simulink model "Quadrotor_model"  (R2018a)
settings: Solver=ode45  StartTime=0.0  StopTime=tSpan  RelTol=1e-3  EnableMultiTasking=on
values from neighbouring files (symbols this model uses):
  a1 = 16.235    [QuadrotorConstants.m]    (also in QuadrotorConstants.mat; TuningParameters.mat)
  a2 = 17.912    [QuadrotorConstants.m]    (also in QuadrotorConstants.mat; TuningParameters.mat)
  a3 = 17.914    [QuadrotorConstants.m]    (also in QuadrotorConstants.mat; TuningParameters.mat)
  a4 = 18.161    [QuadrotorConstants.m]    (also in QuadrotorConstants.mat; TuningParameters.mat)
  angSatLimit = 250    [QuadrotorConstants.m]    (also in QuadrotorConstants.mat; TuningParameters.mat)
  b1 = -0.5036    [QuadrotorConstants.m]    (also in QuadrotorConstants.mat; TuningParameters.mat)
  b2 = -12.728    [QuadrotorConstants.m]    (also in QuadrotorConstants.mat; TuningParameters.mat)
  b3 = -6.5646    [QuadrotorConstants.m]    (also in QuadrotorConstants.mat; TuningParameters.mat)
  b4 = -7.4637    [QuadrotorConstants.m]    (also in QuadrotorConstants.mat; TuningParameters.mat)
  bb = 2.6846e-07    [QuadrotorConstants.m]    (also in QuadrotorConstants.mat; TuningParameters.mat)
  c = 0.0002    [QuadrotorConstants.m]    (also in QuadrotorConstants.mat; TuningParameters.mat)
  c_mi_x = 1.70    (= 1.7)    [QuadrotorConstants.m]    (also in QuadrotorConstants.mat; TuningParameters.mat)
  c_mi_y = 1.70    (= 1.7)    [QuadrotorConstants.m]    (also in QuadrotorConstants.mat; TuningParameters.mat)
  c_mi_z = 0.40    (= 0.4)    [QuadrotorConstants.m]    (also in QuadrotorConstants.mat; TuningParameters.mat)
  co_x = 1.7    [QuadrotorConstants.m]    (also in QuadrotorConstants.mat; TuningParameters.mat)
  co_y = 1.7    [QuadrotorConstants.m]    (also in QuadrotorConstants.mat; TuningParameters.mat)
  co_z = 3    [QuadrotorConstants.m]    (also in QuadrotorConstants.mat; TuningParameters.mat)
  d = 0.0071    [QuadrotorConstants.m]    (also in QuadrotorConstants.mat; TuningParameters.mat)
  d_omega_R10 = V1_WP    [InitialConditions.m]    (also in TuningParameters.mat = 0.286149195881)
  d_omega_R20 = V2_WP    [InitialConditions.m]    (also in TuningParameters.mat = 0.941828505757)
  d_omega_R30 = V3_WP    [InitialConditions.m]    (also in TuningParameters.mat = 0.597668426656)
  d_omega_R40 = V4_WP    [InitialConditions.m]    (also in TuningParameters.mat = 0.639046979523)
  dd = 2.4481e-03    (= 0.0024481)    [QuadrotorConstants.m]    (also in QuadrotorConstants.mat; TuningParameters.mat)
  dfi_0 = 0    [InitialConditions.m]    (also in TuningParameters.mat)
  disturbancePhi = 0    [runMain.m]
  disturbancePsi = 0    [runMain.m]
  disturbanceTheta = 0    [runMain.m]
  disturbancex = 0    [runMain.m]
  disturbancey = 0    [runMain.m]
  disturbancez = 0    [runMain.m]
  dpsi_0 = 0    [InitialConditions.m]    (also in TuningParameters.mat)
  dtheta_0 = 0    [InitialConditions.m]    (also in TuningParameters.mat)
  dx_0 = 0    [InitialConditions.m]    (also in TuningParameters.mat)
  dy_0 = 0    [InitialConditions.m]    (also in TuningParameters.mat)
  dz_0 = 5    [InitialConditions.m]    (also in TuningParameters.mat)
  f = 5e-6    (= 5e-06)    [QuadrotorConstants.m]    (also in QuadrotorConstants.mat; TuningParameters.mat; animateQuadrotor.m = getframe; animateQuadrotorConstant.m = getframe)
  fi_0 = pi    (= 3.14159265359)    [InitialConditions.m]    (also in TuningParameters.mat)
  g = 0.0008    [QuadrotorConstants.m]    (also in QuadrotorConstants.mat; TuningParameters.mat)
  ga = 9.807    [QuadrotorConstants.m]    (also in QuadrotorConstants.mat; TuningParameters.mat)
  h = -0.0282    [QuadrotorConstants.m]    (also in QuadrotorConstants.mat; TuningParameters.mat)
  Ixx = 2.1385*1    (= 2.1385)    [QuadrotorConstants.m]    (also in QuadrotorConstants.mat; TuningParameters.mat)
  Iyy = Ixx    (= 2.1385)    [QuadrotorConstants.m]    (also in QuadrotorConstants.mat; TuningParameters.mat)
  Izz = 3.7479*1    (= 3.7479)    [QuadrotorConstants.m]    (also in QuadrotorConstants.mat; TuningParameters.mat)
  Jr = 4.86851*0.1    (= 0.486851)    [QuadrotorConstants.m]    (also in QuadrotorConstants.mat; TuningParameters.mat)
  L = 0.422    [QuadrotorConstants.m]    (also in QuadrotorConstants.mat; TuningParameters.mat)
  lambda_phi = 50/kd_phi    (= 5)    [TuningParameters.m]    (also in TuningParameters.mat)
  lambda_psi = 50/kd_psi    (= 5)    [TuningParameters.m]    (also in TuningParameters.mat)
  lambda_theta = 50/kd_theta    (= 5)    [TuningParameters.m]    (also in TuningParameters.mat)
  lambda_z = 50/kd_z    (= 5)    [TuningParameters.m]    (also in TuningParameters.mat)
  m = 2.1    [QuadrotorConstants.m]    (also in QuadrotorConstants.mat; TuningParameters.mat)
  psi_0 = 0    [InitialConditions.m]    (also in TuningParameters.mat)
  Tau = 0.1    [QuadrotorConstants.m]    (also in QuadrotorConstants.mat; TuningParameters.mat)
  theta_0 = 0    [InitialConditions.m]    (also in TuningParameters.mat)
  x_0 = 0    [InitialConditions.m]    (also in TuningParameters.mat)
  y_0 = 0    [InitialConditions.m]    (also in TuningParameters.mat)
  z_0 = 10    [InitialConditions.m]    (also in TuningParameters.mat)
undefined symbols (not defined in the file or in its folder): sigbuilder_block
settings Model: Creator=Jake  LastModifiedBy=mdom9
settings DataIOCC: LimitDataPoints=on  SaveFormat=Array  SignalLoggingSaveFormat=ModelDataLogs
settings OptimizationCC: InitFltsAndDblsToZero=on  LifeSpan=inf
settings DebuggingCC: SaveWithParameterizedLinksMsg=none  UnderspecifiedInitializationDetection=Classic  MergeDetectMultiDrivingBlocksExec=none  SignalResolutionControl=TryResolveAllWithWarning  MultiTaskDSMMsg=warning  MultiTaskCondExecSysMsg=none  FcnCallInpInsideContextMsg=warning  SFUnexpectedBacktrackingDiag=warning  SFNoUnconditionalDefaultTransitionDiag=warning  SFExecutionAtInitializationDiag=none
settings HardwareCC: ProdBitPerPointer=32  ProdBitPerSizeT=32  ProdBitPerPtrDiffT=32  ProdLargestAtomicFloat=None  ProdIntDivRoundTo=Undefined  ProdEndianess=Unspecified  ProdWordSize=32  ProdHWDeviceType=32-bit Generic
settings ModelReferenceCC: PropagateSignalLabelsOutOfModel=off
settings SFSimCC: SimParseCustomCode=off
settings CodeAppCC: StateflowObjectComments=on
settings GRTTargetCC: TargetFcnLib=ansi_tfl_tmw.mat  TargetLangStandard=C89/C90 (ANSI)  CombineOutputUpdateFcns=off  GRTInterface=on
settings ConfigComp: CovMetricSettings=dw  CovHtmlReporting=on  CovSaveCumulativeToWorkspaceVar=on  CovSaveSingleToWorkspaceVar=on  CovExternalEMLEnable=off
settings SimscapeCC: SimscapeNormalizeSystem=off

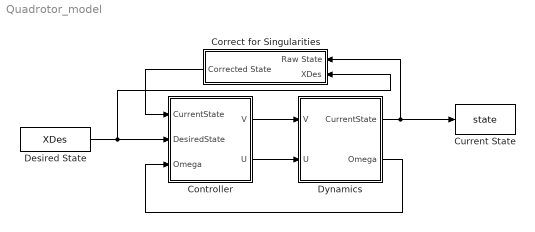
== system Quadrotor_model ==
  Controller : Subsystem
  Correct for Singularities : Subsystem
  Current State : ToWorkspace  VariableName=state  SaveFormat=Timeseries  SampleTime=-1
  Desired State : FromWorkspace  VariableName=XDes  SampleTime=0
  Dynamics : Subsystem
  wires:
  Controller/1(V) -> Dynamics/1(V)
  Dynamics/2(Omega) -> Controller/3(Omega)
  Dynamics/1("CurrentState ") -> Current State/1, Correct for Singularities/1(Raw State)
  Controller/2(U) -> Dynamics/2(U)
  Desired State/1 -> Correct for Singularities/2(XDes), Controller/2(DesiredState)
  Correct for Singularities/1(Corrected State) -> Controller/1("CurrentState ")

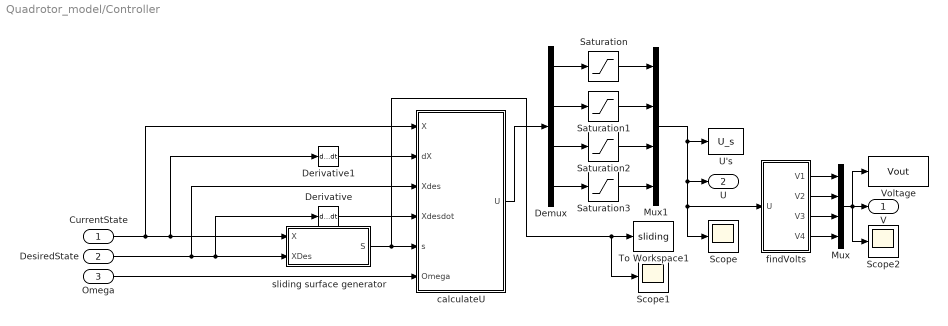
== system Quadrotor_model/Controller ==
  "CurrentState " : Inport
  DesiredState : Inport  Port=2
  Omega : Inport  Port=3
  Demux : Demux
  Derivative : Derivative
  Derivative1 : Derivative
  Mux : Mux
  Mux1 : Mux
  Saturation : Saturate  UpperLimit=60  LowerLimit=0
  Saturation1 : Saturate  UpperLimit=angSatLimit  LowerLimit=-angSatLimit
  Saturation2 : Saturate  UpperLimit=angSatLimit  LowerLimit=-angSatLimit
  Saturation3 : Saturate  UpperLimit=angSatLimit  LowerLimit=-angSatLimit
  Scope : Scope
  Scope1 : Scope
  Scope2 : Scope
  To Workspace1 : ToWorkspace  VariableName=sliding  SaveFormat=Timeseries  SampleTime=-1
  U's : ToWorkspace  VariableName=U_s  SaveFormat=Timeseries  SampleTime=-1
  Voltage : ToWorkspace  VariableName=Vout  SaveFormat=Timeseries  SampleTime=-1
  calculateU : MATLAB Function  TreatAsAtomicUnit=on
  findVolts : Subsystem
  sliding surface generator : Subsystem
  V : Outport
  U : Outport  Port=2
  wires:
  sliding surface generator/1(S) -> calculateU/5(s), Scope1/1, To Workspace1/1
  findVolts/1(V1) -> Mux/1
  findVolts/2(V2) -> Mux/2
  findVolts/3(V3) -> Mux/3
  findVolts/4(V4) -> Mux/4
  Mux/1 -> Voltage/1, Scope2/1, V/1
  Omega/1 -> calculateU/6(Omega)
  "CurrentState "/1 -> calculateU/1(X), Derivative1/1, sliding surface generator/1(X)
  DesiredState/1 -> calculateU/3(Xdes), Derivative/1, sliding surface generator/2(XDes)
  Derivative/1 -> calculateU/4(Xdesdot)
  Derivative1/1 -> calculateU/2(dX)
  Mux1/1 -> Scope/1, findVolts/1(U), U/1, U's/1
  Demux/1 -> Saturation/1
  Demux/2 -> Saturation1/1
  Demux/3 -> Saturation2/1
  Demux/4 -> Saturation3/1
  calculateU/1(U) -> Demux/1
  Saturation/1 -> Mux1/1
  Saturation1/1 -> Mux1/2
  Saturation2/1 -> Mux1/3
  Saturation3/1 -> Mux1/4

== system Quadrotor_model/Correct for Singularities ==
  Raw State : Inport
  XDes : Inport  Port=2
  "Check for singularity in phi, theta" : Subsystem
  DIsplay Uncorrected State : Subsystem
  Display Corrected State : Subsystem
  Corrected State : Outport
  wires:
  Raw State/1 -> "Check for singularity in phi, theta"/1(Current State), DIsplay Uncorrected State/1(Uncorrected State)
  "Check for singularity in phi, theta"/1("Correct State ") -> Corrected State/1, Display Corrected State/1(Corrected State)
  XDes/1 -> "Check for singularity in phi, theta"/2(XDes)

== system Quadrotor_model/Dynamics ==
  V : Inport
  U : Inport  Port=2
  Body dynamics : Subsystem
  Demux : Demux
  Demux1 : Demux
  Motor dynamics : Subsystem
  Mux : Mux  Inputs=2
  "CurrentState " : Outport
  Omega : Outport  Port=2
  wires:
  Mux/1 -> "CurrentState "/1
  V/1 -> Demux/1
  Demux/1 -> Motor dynamics/1(V1)
  Demux/2 -> Motor dynamics/2(V2)
  Demux/3 -> Motor dynamics/3(V3)
  Demux/4 -> Motor dynamics/4(V4)
  Motor dynamics/1(Omega) -> Omega/1, Body dynamics/5(Omega)
  Demux1/1 -> Body dynamics/1(U1)
  Demux1/2 -> Body dynamics/2(U2)
  Demux1/3 -> Body dynamics/3(U3)
  Demux1/4 -> Body dynamics/4(U4)
  U/1 -> Demux1/1
  Body dynamics/1(Position) -> Mux/1
  Body dynamics/2(Orientation) -> Mux/2

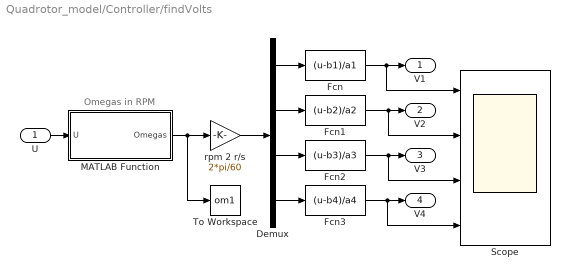
== system Quadrotor_model/Controller/findVolts ==
  note: Omegas in RPM
  U : Inport
  Demux : Demux
  Fcn : Fcn  Expr=(u-b1)/a1
  Fcn1 : Fcn  Expr=(u-b2)/a2
  Fcn2 : Fcn  Expr=(u-b3)/a3
  Fcn3 : Fcn  Expr=(u-b4)/a4
  MATLAB Function : MATLAB Function  TreatAsAtomicUnit=on
  Scope : Scope  NumInputPorts=4
  To Workspace : ToWorkspace  VariableName=om1  SaveFormat=Timeseries  SampleTime=-1
  rpm 2 r/s : Gain  Gain=2*pi/60
  V1 : Outport
  V2 : Outport  Port=2
  V3 : Outport  Port=3
  V4 : Outport  Port=4
  wires:
  Fcn3/1 -> Scope/4, V4/1
  Fcn2/1 -> Scope/3, V3/1
  Fcn1/1 -> Scope/2, V2/1
  Fcn/1 -> Scope/1, V1/1
  Demux/1 -> Fcn/1
  Demux/3 -> Fcn2/1
  Demux/2 -> Fcn1/1
  rpm 2 r/s/1 -> Demux/1
  Demux/4 -> Fcn3/1
  MATLAB Function/1(Omegas) -> To Workspace/1, rpm 2 r/s/1
  U/1 -> MATLAB Function/1(U)

== system Quadrotor_model/Controller/sliding surface generator ==
  X : Inport
  XDes : Inport  Port=2
  Add : Sum  Inputs=+++
  Derivative : Derivative
  Gain : Gain  Gain=[lambda_z lambda_phi lambda_theta lambda_psi].'
  Integrator : Integrator
  Scope : Scope
  Selector : Selector  InputPortWidth=12  IndexOptions=Index vector (dialog)  Indices=[5 7 9 11]  OutputSizes=1
  error : Sum  Inputs=-+
  S : Outport
  wires:
  Gain/1 -> Add/1
  error/1 -> Scope/1, Selector/1
  Add/1 -> S/1
  Derivative/1 -> Add/2
  Integrator/1 -> Add/3
  Selector/1 -> Integrator/1, Gain/1, Derivative/1
  X/1 -> error/1
  XDes/1 -> error/2

== system Quadrotor_model/Correct for Singularities/Check for singularity in phi, theta ==
  Current State : Inport
  XDes : Inport  Port=2
  Singularity in phi : Subsystem
  Singularity in theta : Subsystem
  "Correct State " : Outport
  wires:
  Singularity in phi/1(Modified State) -> Singularity in theta/1(Current State)
  Singularity in theta/1(Modified State) -> "Correct State "/1
  Current State/1 -> Singularity in phi/1(Current State)
  XDes/1 -> Singularity in phi/2(XDes), Singularity in theta/2(XDes)

== system Quadrotor_model/Correct for Singularities/DIsplay Uncorrected State ==
  Uncorrected State : Inport
  Constant : Constant  Value=0
  Scope1 : Scope
  Selector2 : Selector  InputPortWidth=12  IndexOptions=Index vector (dialog)  Indices=[7 9]  OutputSizes=1
  Subtract : Sum  Inputs=+-
  To Workspace1 : ToWorkspace  VariableName=rawAngles  SaveFormat=Timeseries  SampleTime=-1
  wires:
  Constant/1 -> Subtract/2
  Selector2/1 -> Subtract/1
  Subtract/1 -> Scope1/1, To Workspace1/1
  Uncorrected State/1 -> Selector2/1

== system Quadrotor_model/Correct for Singularities/Display Corrected State ==
  Corrected State : Inport
  Constant1 : Constant  Value=0
  Scope2 : Scope
  Selector1 : Selector  InputPortWidth=12  IndexOptions=Index vector (dialog)  Indices=[7 9]  OutputSizes=1
  Subtract1 : Sum  Inputs=+-
  To Workspace : ToWorkspace  VariableName=correctedAngles  SaveFormat=Timeseries  SampleTime=-1
  wires:
  Constant1/1 -> Subtract1/2
  Subtract1/1 -> To Workspace/1, Scope2/1
  Selector1/1 -> Subtract1/1
  Corrected State/1 -> Selector1/1

== system Quadrotor_model/Dynamics/Body dynamics ==
  U1 : Inport
  U2 : Inport  Port=2
  U3 : Inport  Port=3
  U4 : Inport  Port=4
  Omega : Inport  Port=5
  Mux : Mux  Inputs=6
  Pitch Stability : Subsystem
  Position Stability : Subsystem
  Roll Stability : Subsystem
  Yaw Stability : Subsystem
  Position : Outport
  Orientation : Outport  Port=2
  wires:
  U4/1 -> Yaw Stability/1(U4)
  U3/1 -> Pitch Stability/3(U3)
  U1/1 -> Position Stability/1(U1)
  U2/1 -> Roll Stability/2(U2)
  Omega/1 -> Pitch Stability/2(SumYRtrSpd), Roll Stability/1(SumXRtrSpd)
  Roll Stability/1(Phi) -> Position Stability/2(fi), Mux/1
  Pitch Stability/1(Theta) -> Position Stability/3(theta), Mux/3
  Yaw Stability/1(Psi) -> Position Stability/4(psi), Mux/5
  Roll Stability/2(dPhi) -> Mux/2, Yaw Stability/2(dPhi), Pitch Stability/1(dPhi)
  Yaw Stability/2(dPsi) -> Roll Stability/4(dPsi), Pitch Stability/4(dPsi), Mux/6
  Pitch Stability/2(dTheta) -> Yaw Stability/3(dTheta), Roll Stability/3(dTheta), Mux/4
  Position Stability/1(Position) -> Position/1
  Mux/1 -> Orientation/1

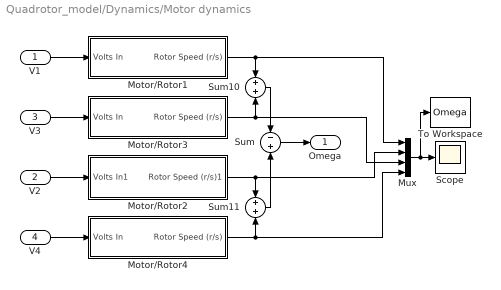
== system Quadrotor_model/Dynamics/Motor dynamics ==
  V1 : Inport
  V2 : Inport  Port=2
  V3 : Inport  Port=3
  V4 : Inport  Port=4
  Motor/Rotor1 : Subsystem
  Motor/Rotor2 : Subsystem
  Motor/Rotor3 : Subsystem
  Motor/Rotor4 : Subsystem
  Mux : Mux
  Scope : Scope
  Sum : Sum  Inputs=-+
  Sum10 : Sum  Inputs=+|+
  Sum11 : Sum  Inputs=+|+
  To Workspace : ToWorkspace  VariableName=Omega  SaveFormat=Timeseries  SampleTime=-1
  Omega : Outport
  wires:
  Sum11/1 -> Sum/2
  Sum10/1 -> Sum/1
  Motor/Rotor4/1(Rotor Speed (r/s)) -> Mux/4, Sum11/2
  Motor/Rotor3/1(Rotor Speed (r/s)) -> Mux/3, Sum10/2
  Motor/Rotor2/1(Rotor Speed (r/s)1) -> Mux/2, Sum11/1
  Motor/Rotor1/1(Rotor Speed (r/s)) -> Mux/1, Sum10/1
  Sum/1 -> Omega/1
  V1/1 -> Motor/Rotor1/1(Volts In)
  V4/1 -> Motor/Rotor4/1(Volts In)
  V3/1 -> Motor/Rotor3/1(Volts In)
  V2/1 -> Motor/Rotor2/1(Volts In1)
  Mux/1 -> To Workspace/1, Scope/1

== system Quadrotor_model/Correct for Singularities/Check for singularity in phi, theta/Singularity in phi ==
  Current State : Inport
  XDes : Inport  Port=2
  CorrectPhi : MATLAB Function  TreatAsAtomicUnit=on
  Modified State : Outport
  wires:
  Current State/1 -> CorrectPhi/1(X)
  CorrectPhi/1(newX) -> Modified State/1
  XDes/1 -> CorrectPhi/2(XDes)

== system Quadrotor_model/Correct for Singularities/Check for singularity in phi, theta/Singularity in theta ==
  Current State : Inport
  XDes : Inport  Port=2
  CorrectTheta : MATLAB Function  TreatAsAtomicUnit=on
  Modified State : Outport
  wires:
  Current State/1 -> CorrectTheta/1(X)
  CorrectTheta/1(newX) -> Modified State/1
  XDes/1 -> CorrectTheta/2(XDes)

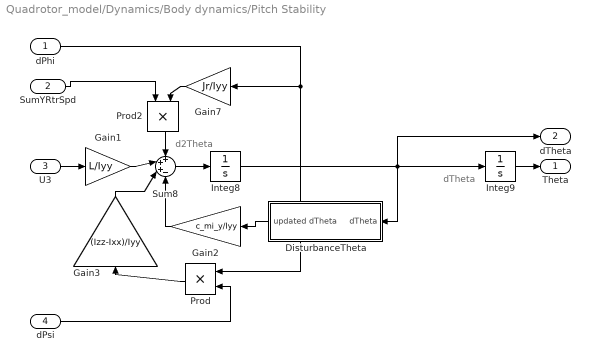
== system Quadrotor_model/Dynamics/Body dynamics/Pitch Stability ==
  note: d2Theta
  note: dTheta
  dPhi : Inport
  SumYRtrSpd : Inport  Port=2
  U3 : Inport  Port=3
  dPsi : Inport  Port=4
  DisturbanceTheta : Subsystem
  Gain1 : Gain  Gain=L/Iyy
  Gain2 : Gain  Gain=c_mi_y/Iyy
  Gain3 : Gain  Gain=(Izz-Ixx)/Iyy
  Gain7 : Gain  Gain=Jr/Iyy
  Integ8 : Integrator  InitialCondition=dtheta_0
  Integ9 : Integrator  InitialCondition=theta_0  UpperSaturationLimit=pi/2  LowerSaturationLimit=-pi/2
  Prod : Product  RndMeth=Zero
  Prod2 : Product  RndMeth=Zero
  Sum8 : Sum  Inputs=+++-
  Theta : Outport
  dTheta : Outport  Port=2
  wires:
  Gain2/1 -> Sum8/4
  dPhi/1 -> Prod/1, Gain7/1
  Integ9/1 -> Theta/1
  U3/1 -> Gain1/1
  SumYRtrSpd/1 -> Prod2/1
  dPsi/1 -> Prod/2
  Integ8/1 -> dTheta/1, DisturbanceTheta/1(dTheta), Integ9/1
  Sum8/1 -> Integ8/1
  Gain1/1 -> Sum8/2
  Gain7/1 -> Prod2/2
  Gain3/1 -> Sum8/3
  Prod/1 -> Gain3/1
  Prod2/1 -> Sum8/1
  DisturbanceTheta/1(updated dTheta) -> Gain2/1

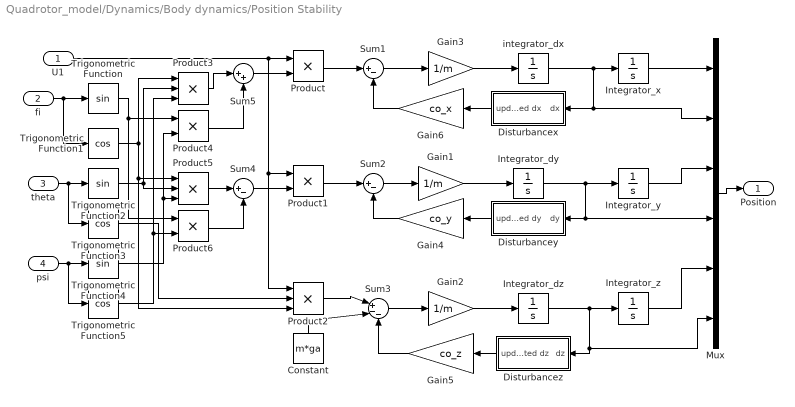
== system Quadrotor_model/Dynamics/Body dynamics/Position Stability ==
  U1 : Inport
  fi : Inport  Port=2
  theta : Inport  Port=3
  psi : Inport  Port=4
  Constant : Constant  Value=m*ga
  Disturbancex : Subsystem
  Disturbancey : Subsystem
  Disturbancez : Subsystem
  Gain1 : Gain  Gain=1/m
  Gain2 : Gain  Gain=1/m
  Gain3 : Gain  Gain=1/m
  Gain4 : Gain  Gain=co_y
  Gain5 : Gain  Gain=co_z
  Gain6 : Gain  Gain=co_x
  Integrator_dy : Integrator  InitialCondition=dy_0  LimitOutput=on  UpperSaturationLimit=1000  LowerSaturationLimit=-1000
  Integrator_dz : Integrator  InitialCondition=dz_0  LimitOutput=on  UpperSaturationLimit=1000  LowerSaturationLimit=-1000
  Integrator_x : Integrator  InitialCondition=x_0
  Integrator_y : Integrator  InitialCondition=y_0
  Integrator_z : Integrator  InitialCondition=z_0
  Mux : Mux  Inputs=6
  Product{,1,4,6} (4 alike) : Product  RndMeth=Zero
  Product2 : Product  Inputs=3  RndMeth=Zero
  Product3 : Product  Inputs=3  RndMeth=Zero
  Product5 : Product  Inputs=3  RndMeth=Zero
  Sum1 : Sum  Inputs=|+-
  Sum2 : Sum  Inputs=|+-
  Sum3 : Sum  Inputs=|+--
  Sum4 : Sum  Inputs=|+-
  Sum5 : Sum  Inputs=|++
  Trigonometric Function : Trigonometry
  Trigonometric Function1 : Trigonometry  Operator=cos
  Trigonometric Function2 : Trigonometry
  Trigonometric Function3 : Trigonometry  Operator=cos
  Trigonometric Function4 : Trigonometry
  Trigonometric Function5 : Trigonometry  Operator=cos
  integrator_dx : Integrator  InitialCondition=dx_0  LimitOutput=on  UpperSaturationLimit=1000  LowerSaturationLimit=-1000
  Position : Outport
  wires:
  Gain5/1 -> Sum3/3
  Constant/1 -> Sum3/2
  Gain4/1 -> Sum2/2
  Sum3/1 -> Gain2/1
  Gain6/1 -> Sum1/2
  Product2/1 -> Sum3/1
  Sum2/1 -> Gain1/1
  Product1/1 -> Sum2/1
  Gain2/1 -> Integrator_dz/1
  Sum1/1 -> Gain3/1
  Product/1 -> Sum1/1
  U1/1 -> Product/1, Product1/1, Product2/1
  Integrator_x/1 -> Mux/1
  integrator_dx/1 -> Integrator_x/1, Disturbancex/1(dx), Mux/2
  Integrator_dy/1 -> Integrator_y/1, Disturbancey/1(dy), Mux/4
  Integrator_dz/1 -> Integrator_z/1, Disturbancez/1(dz), Mux/6
  Gain1/1 -> Integrator_dy/1
  Gain3/1 -> integrator_dx/1
  Sum4/1 -> Product1/2
  Sum5/1 -> Product/2
  Product3/1 -> Sum5/1
  Product4/1 -> Sum5/2
  Product5/1 -> Sum4/1
  Product6/1 -> Sum4/2
  psi/1 -> Trigonometric Function4/1, Trigonometric Function5/1
  theta/1 -> Trigonometric Function2/1, Trigonometric Function3/1
  fi/1 -> Trigonometric Function/1, Trigonometric Function1/1
  Trigonometric Function/1 -> Product4/1, Product6/1
  Trigonometric Function1/1 -> Product3/1, Product5/1, Product2/3
  Trigonometric Function2/1 -> Product3/2, Product5/2
  Trigonometric Function5/1 -> Product3/3, Product6/2
  Trigonometric Function4/1 -> Product4/2, Product5/3
  Trigonometric Function3/1 -> Product2/2
  Integrator_y/1 -> Mux/3
  Integrator_z/1 -> Mux/5
  Mux/1 -> Position/1
  Disturbancez/1(updated dz) -> Gain5/1
  Disturbancey/1(updated dy) -> Gain4/1
  Disturbancex/1(updated dx) -> Gain6/1

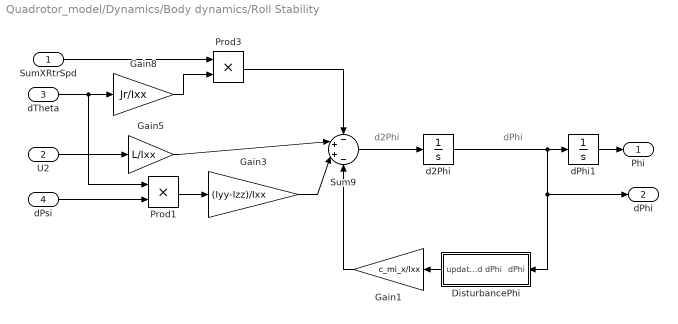
== system Quadrotor_model/Dynamics/Body dynamics/Roll Stability ==
  note: d2Phi
  note: dPhi
  SumXRtrSpd : Inport
  U2 : Inport  Port=2
  dTheta : Inport  Port=3
  dPsi : Inport  Port=4
  DisturbancePhi : Subsystem
  Gain1 : Gain  Gain=c_mi_x/Ixx
  Gain3 : Gain  Gain=(Iyy-Izz)/Ixx
  Gain5 : Gain  Gain=L/Ixx
  Gain8 : Gain  Gain=Jr/Ixx
  Prod1 : Product  RndMeth=Zero
  Prod3 : Product  RndMeth=Zero
  Sum9 : Sum  Inputs=-++-
  d2Phi : Integrator  InitialCondition=dfi_0
  dPhi1 : Integrator  InitialCondition=fi_0  UpperSaturationLimit=pi/2  LowerSaturationLimit=-pi/2
  Phi : Outport
  dPhi : Outport  Port=2
  wires:
  dPsi/1 -> Prod1/2
  dTheta/1 -> Prod1/1, Gain8/1
  Prod3/1 -> Sum9/1
  SumXRtrSpd/1 -> Prod3/1
  Gain8/1 -> Prod3/2
  dPhi1/1 -> Phi/1
  U2/1 -> Gain5/1
  d2Phi/1 -> DisturbancePhi/1(dPhi), dPhi/1, dPhi1/1
  Sum9/1 -> d2Phi/1
  Gain5/1 -> Sum9/2
  Gain1/1 -> Sum9/4
  Gain3/1 -> Sum9/3
  Prod1/1 -> Gain3/1
  DisturbancePhi/1(updated dPhi) -> Gain1/1

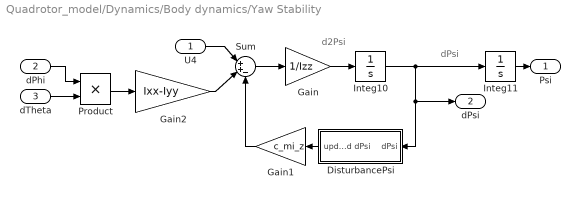
== system Quadrotor_model/Dynamics/Body dynamics/Yaw Stability ==
  note: dPsi
  note: d2Psi
  U4 : Inport
  dPhi : Inport  Port=2
  dTheta : Inport  Port=3
  DisturbancePsi : Subsystem
  Gain : Gain  Gain=1/Izz
  Gain1 : Gain  Gain=c_mi_z
  Gain2 : Gain  Gain=Ixx-Iyy
  Integ10 : Integrator  InitialCondition=dpsi_0
  Integ11 : Integrator  InitialCondition=psi_0
  Product : Product  RndMeth=Zero
  Sum : Sum  Inputs=|++-
  Psi : Outport
  dPsi : Outport  Port=2
  wires:
  Sum/1 -> Gain/1
  U4/1 -> Sum/1
  Integ11/1 -> Psi/1
  Gain/1 -> Integ10/1
  Integ10/1 -> DisturbancePsi/1(dPsi), dPsi/1, Integ11/1
  Gain1/1 -> Sum/3
  Gain2/1 -> Sum/2
  dPhi/1 -> Product/1
  dTheta/1 -> Product/2
  Product/1 -> Gain2/1
  DisturbancePsi/1(updated dPsi) -> Gain1/1

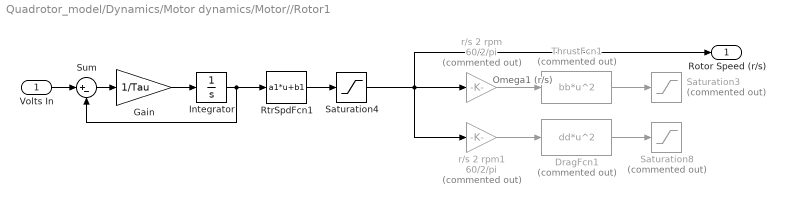
== system Quadrotor_model/Dynamics/Motor dynamics/Motor//Rotor1 ==
  note: Omega1
      | (r/s)
  Volts In : Inport
  DragFcn1 : Fcn  Commented=on  Expr=dd*u^2
  Gain : Gain  Gain=1/Tau
  Integrator : Integrator  InitialCondition=d_omega_R10
  RtrSpdFcn1 : Fcn  Expr=a1*u+b1
  Saturation3 : Saturate  Commented=on  UpperLimit=1000  LowerLimit=-1000
  Saturation4 : Saturate  UpperLimit=250  LowerLimit=0
  Saturation8 : Saturate  Commented=on  UpperLimit=1000  LowerLimit=-1000
  Sum : Sum  Inputs=|+-
  ThrustFcn1 : Fcn  Commented=on  Expr=bb*u^2
  r/s 2 rpm : Gain  Commented=on  Gain=60/2/pi
  r/s 2 rpm1 : Gain  Commented=on  Gain=60/2/pi
  Rotor Speed (r/s) : Outport
  wires:
  Volts In/1 -> Sum/1
  Sum/1 -> Gain/1
  Integrator/1 -> RtrSpdFcn1/1, Sum/2
  Gain/1 -> Integrator/1
  DragFcn1/1 -> Saturation8/1
  RtrSpdFcn1/1 -> Saturation4/1
  ThrustFcn1/1 -> Saturation3/1
  Saturation4/1 -> Rotor Speed (r/s)/1, r/s 2 rpm1/1, r/s 2 rpm/1
  r/s 2 rpm/1 -> ThrustFcn1/1
  r/s 2 rpm1/1 -> DragFcn1/1

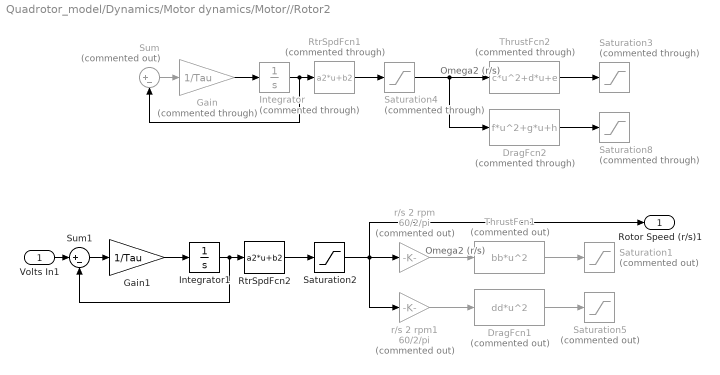
== system Quadrotor_model/Dynamics/Motor dynamics/Motor//Rotor2 ==
  note: Omega2
      | (r/s)
  note: Omega2
      | (r/s)
  Volts In1 : Inport
  DragFcn1 : Fcn  Commented=on  Expr=dd*u^2
  DragFcn2 : Fcn  Commented=through  Expr=f*u^2+g*u+h
  Gain : Gain  Commented=through  Gain=1/Tau
  Gain1 : Gain  Gain=1/Tau
  Integrator : Integrator  Commented=through  InitialCondition=d_omega_R20
  Integrator1 : Integrator  InitialCondition=d_omega_R20
  RtrSpdFcn1 : Fcn  Commented=through  Expr=a2*u+b2
  RtrSpdFcn2 : Fcn  Expr=a2*u+b2
  Saturation1 : Saturate  Commented=on  UpperLimit=1000  LowerLimit=-1000
  Saturation2 : Saturate  UpperLimit=250  LowerLimit=0
  Saturation3 : Saturate  Commented=through  UpperLimit=1000  LowerLimit=-1000
  Saturation4 : Saturate  Commented=through  UpperLimit=1000  LowerLimit=-1000
  Saturation5 : Saturate  Commented=on  UpperLimit=1000  LowerLimit=-1000
  Saturation8 : Saturate  Commented=through  UpperLimit=1000  LowerLimit=-1000
  Sum : Sum  Commented=on  Inputs=|+-
  Sum1 : Sum  Inputs=|+-
  ThrustFcn1 : Fcn  Commented=on  Expr=bb*u^2
  ThrustFcn2 : Fcn  Commented=through  Expr=c*u^2+d*u+e
  r/s 2 rpm : Gain  Commented=on  Gain=60/2/pi
  r/s 2 rpm1 : Gain  Commented=on  Gain=60/2/pi
  Rotor Speed (r/s)1 : Outport
  wires:
  Sum/1 -> Gain/1
  Integrator/1 -> RtrSpdFcn1/1, Sum/2
  Gain/1 -> Integrator/1
  RtrSpdFcn1/1 -> Saturation4/1
  ThrustFcn2/1 -> Saturation3/1
  Saturation4/1 -> DragFcn2/1, ThrustFcn2/1
  DragFcn2/1 -> Saturation8/1
  DragFcn1/1 -> Saturation5/1
  Integrator1/1 -> RtrSpdFcn2/1, Sum1/2
  Gain1/1 -> Integrator1/1
  RtrSpdFcn2/1 -> Saturation2/1
  ThrustFcn1/1 -> Saturation1/1
  Volts In1/1 -> Sum1/1
  Sum1/1 -> Gain1/1
  Saturation2/1 -> Rotor Speed (r/s)1/1, r/s 2 rpm1/1, r/s 2 rpm/1
  r/s 2 rpm1/1 -> DragFcn1/1
  r/s 2 rpm/1 -> ThrustFcn1/1

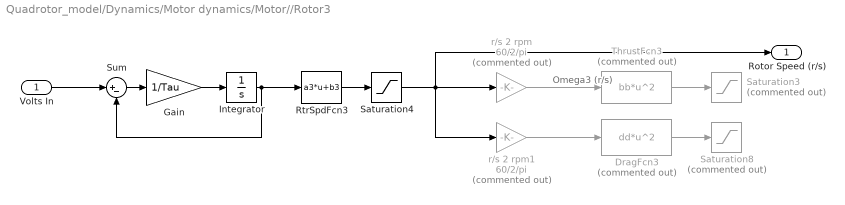
== system Quadrotor_model/Dynamics/Motor dynamics/Motor//Rotor3 ==
  note: Omega3
      | (r/s)
  Volts In : Inport
  DragFcn3 : Fcn  Commented=on  Expr=dd*u^2
  Gain : Gain  Gain=1/Tau
  Integrator : Integrator  InitialCondition=d_omega_R30
  RtrSpdFcn3 : Fcn  Expr=a3*u+b3
  Saturation3 : Saturate  Commented=on  UpperLimit=1000  LowerLimit=-1000
  Saturation4 : Saturate  UpperLimit=250  LowerLimit=0
  Saturation8 : Saturate  Commented=on  UpperLimit=1000  LowerLimit=-1000
  Sum : Sum  Inputs=|+-
  ThrustFcn3 : Fcn  Commented=on  Expr=bb*u^2
  r/s 2 rpm : Gain  Commented=on  Gain=60/2/pi
  r/s 2 rpm1 : Gain  Commented=on  Gain=60/2/pi
  Rotor Speed (r/s) : Outport
  wires:
  Volts In/1 -> Sum/1
  Sum/1 -> Gain/1
  Integrator/1 -> RtrSpdFcn3/1, Sum/2
  Gain/1 -> Integrator/1
  RtrSpdFcn3/1 -> Saturation4/1
  ThrustFcn3/1 -> Saturation3/1
  DragFcn3/1 -> Saturation8/1
  Saturation4/1 -> Rotor Speed (r/s)/1, r/s 2 rpm1/1, r/s 2 rpm/1
  r/s 2 rpm/1 -> ThrustFcn3/1
  r/s 2 rpm1/1 -> DragFcn3/1

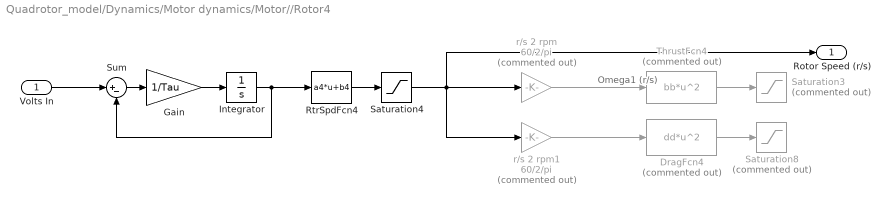
== system Quadrotor_model/Dynamics/Motor dynamics/Motor//Rotor4 ==
  note: Omega1
      | (r/s)
  Volts In : Inport
  DragFcn4 : Fcn  Commented=on  Expr=dd*u^2
  Gain : Gain  Gain=1/Tau
  Integrator : Integrator  InitialCondition=d_omega_R40
  RtrSpdFcn4 : Fcn  Expr=a4*u+b4
  Saturation3 : Saturate  Commented=on  UpperLimit=1000  LowerLimit=-1000
  Saturation4 : Saturate  UpperLimit=250  LowerLimit=0
  Saturation8 : Saturate  Commented=on  UpperLimit=1000  LowerLimit=-1000
  Sum : Sum  Inputs=|+-
  ThrustFcn4 : Fcn  Commented=on  Expr=bb*u^2
  r/s 2 rpm : Gain  Commented=on  Gain=60/2/pi
  r/s 2 rpm1 : Gain  Commented=on  Gain=60/2/pi
  Rotor Speed (r/s) : Outport
  wires:
  Volts In/1 -> Sum/1
  Sum/1 -> Gain/1
  Integrator/1 -> RtrSpdFcn4/1, Sum/2
  Gain/1 -> Integrator/1
  RtrSpdFcn4/1 -> Saturation4/1
  ThrustFcn4/1 -> Saturation3/1
  DragFcn4/1 -> Saturation8/1
  Saturation4/1 -> Rotor Speed (r/s)/1, r/s 2 rpm1/1, r/s 2 rpm/1
  r/s 2 rpm/1 -> ThrustFcn4/1
  r/s 2 rpm1/1 -> DragFcn4/1

== system Quadrotor_model/Dynamics/Body dynamics/Pitch Stability/DisturbanceTheta ==
  dTheta : Inport
  Constant1 : Constant  Value=disturbanceTheta
  If : If  IfExpression=u1 == 1
  If Action Subsystem : Subsystem  TreatAsAtomicUnit=on
  If Action Subsystem1 : Subsystem  TreatAsAtomicUnit=on
  Merge : Merge
  updated dTheta : Outport
  wires:
  If Action Subsystem/1(updated dTheta) -> Merge/1
  If Action Subsystem1/1(updated dTheta) -> Merge/2
  Merge/1 -> updated dTheta/1
  If/2 -> If Action Subsystem1/Action
  Constant1/1 -> If/1
  If/1 -> If Action Subsystem/Action
  dTheta/1 -> If Action Subsystem/1(dTheta), If Action Subsystem1/1(dTheta)

== system Quadrotor_model/Dynamics/Body dynamics/Position Stability/Disturbancex ==
  dx : Inport
  Constant1 : Constant  Value=disturbancex
  If : If  IfExpression=u1 == 1
  If Action Subsystem : Subsystem  TreatAsAtomicUnit=on
  If Action Subsystem1 : Subsystem  TreatAsAtomicUnit=on
  Merge : Merge
  updated dx : Outport
  wires:
  If Action Subsystem/1(updated dx) -> Merge/1
  If Action Subsystem1/1(updated dx) -> Merge/2
  Merge/1 -> updated dx/1
  If/2 -> If Action Subsystem1/Action
  Constant1/1 -> If/1
  If/1 -> If Action Subsystem/Action
  dx/1 -> If Action Subsystem/1(dx), If Action Subsystem1/1(dx)

== system Quadrotor_model/Dynamics/Body dynamics/Position Stability/Disturbancey ==
  dy : Inport
  Constant1 : Constant  Value=disturbancey
  If : If  IfExpression=u1 == 1
  If Action Subsystem : Subsystem  TreatAsAtomicUnit=on
  If Action Subsystem1 : Subsystem  TreatAsAtomicUnit=on
  Merge : Merge
  updated dy : Outport
  wires:
  If Action Subsystem/1(updated dy) -> Merge/1
  If Action Subsystem1/1(updated dy) -> Merge/2
  Merge/1 -> updated dy/1
  If/2 -> If Action Subsystem1/Action
  Constant1/1 -> If/1
  If/1 -> If Action Subsystem/Action
  dy/1 -> If Action Subsystem/1(dy), If Action Subsystem1/1(dy)

== system Quadrotor_model/Dynamics/Body dynamics/Position Stability/Disturbancez ==
  dz : Inport
  Constant1 : Constant  Value=disturbancez
  If : If  IfExpression=u1 == 1
  If Action Subsystem : Subsystem  TreatAsAtomicUnit=on
  If Action Subsystem1 : Subsystem  TreatAsAtomicUnit=on
  Merge : Merge
  updated dz : Outport
  wires:
  If Action Subsystem/1(updated dz) -> Merge/1
  If Action Subsystem1/1(updated dz) -> Merge/2
  Merge/1 -> updated dz/1
  If/2 -> If Action Subsystem1/Action
  Constant1/1 -> If/1
  If/1 -> If Action Subsystem/Action
  dz/1 -> If Action Subsystem/1(dz), If Action Subsystem1/1(dz)

== system Quadrotor_model/Dynamics/Body dynamics/Roll Stability/DisturbancePhi ==
  dPhi : Inport
  Constant1 : Constant  Value=disturbancePhi
  If : If  IfExpression=u1 == 1
  If Action Subsystem : Subsystem  TreatAsAtomicUnit=on
  If Action Subsystem1 : Subsystem  TreatAsAtomicUnit=on
  Merge : Merge
  updated dPhi : Outport
  wires:
  If Action Subsystem/1(updated dPhi) -> Merge/1
  If Action Subsystem1/1(updated dPhi) -> Merge/2
  Merge/1 -> updated dPhi/1
  If/2 -> If Action Subsystem1/Action
  Constant1/1 -> If/1
  If/1 -> If Action Subsystem/Action
  dPhi/1 -> If Action Subsystem/1(dPhi), If Action Subsystem1/1(dPhi)

== system Quadrotor_model/Dynamics/Body dynamics/Yaw Stability/DisturbancePsi ==
  dPsi : Inport
  Constant1 : Constant  Value=disturbancePsi
  If : If  IfExpression=u1 == 1
  If Action Subsystem : Subsystem  TreatAsAtomicUnit=on
  If Action Subsystem1 : Subsystem  TreatAsAtomicUnit=on
  Merge : Merge
  updated dPsi : Outport
  wires:
  If Action Subsystem/1(updated dPsi) -> Merge/1
  If Action Subsystem1/1(updated dPsi) -> Merge/2
  Merge/1 -> updated dPsi/1
  If/2 -> If Action Subsystem1/Action
  Constant1/1 -> If/1
  If/1 -> If Action Subsystem/Action
  dPsi/1 -> If Action Subsystem/1(dPsi), If Action Subsystem1/1(dPsi)

== system Quadrotor_model/Dynamics/Body dynamics/Pitch Stability/DisturbanceTheta/If Action Subsystem ==
  dTheta : Inport
  Action Port : ActionPort  ActionType=then
  add disturbance : Subsystem
  updated dTheta : Outport
  wires:
  dTheta/1 -> add disturbance/1(dTheta)
  add disturbance/1(updated dTheta) -> updated dTheta/1

== system Quadrotor_model/Dynamics/Body dynamics/Pitch Stability/DisturbanceTheta/If Action Subsystem1 ==
  dTheta : Inport
  Action Port : ActionPort  ActionType=else
  updated dTheta : Outport
  wires:
  dTheta/1 -> updated dTheta/1

== system Quadrotor_model/Dynamics/Body dynamics/Position Stability/Disturbancex/If Action Subsystem ==
  dx : Inport
  Action Port : ActionPort  ActionType=then
  add disturbance : Subsystem
  updated dx : Outport
  wires:
  dx/1 -> add disturbance/1(dx)
  add disturbance/1(updated dx) -> updated dx/1

== system Quadrotor_model/Dynamics/Body dynamics/Position Stability/Disturbancex/If Action Subsystem1 ==
  dx : Inport
  Action Port : ActionPort  ActionType=else
  updated dx : Outport
  wires:
  dx/1 -> updated dx/1

== system Quadrotor_model/Dynamics/Body dynamics/Position Stability/Disturbancey/If Action Subsystem ==
  dy : Inport
  Action Port : ActionPort  ActionType=then
  add disturbance : Subsystem
  updated dy : Outport
  wires:
  dy/1 -> add disturbance/1(dy)
  add disturbance/1(updated dy) -> updated dy/1

== system Quadrotor_model/Dynamics/Body dynamics/Position Stability/Disturbancey/If Action Subsystem1 ==
  dy : Inport
  Action Port : ActionPort  ActionType=else
  updated dy : Outport
  wires:
  dy/1 -> updated dy/1

== system Quadrotor_model/Dynamics/Body dynamics/Position Stability/Disturbancez/If Action Subsystem ==
  dz : Inport
  Action Port : ActionPort  ActionType=then
  add disturbance : Subsystem
  updated dz : Outport
  wires:
  dz/1 -> add disturbance/1(dz)
  add disturbance/1(updated dz) -> updated dz/1

== system Quadrotor_model/Dynamics/Body dynamics/Position Stability/Disturbancez/If Action Subsystem1 ==
  dz : Inport
  Action Port : ActionPort  ActionType=else
  updated dz : Outport
  wires:
  dz/1 -> updated dz/1

== system Quadrotor_model/Dynamics/Body dynamics/Roll Stability/DisturbancePhi/If Action Subsystem ==
  dPhi : Inport
  Action Port : ActionPort  ActionType=then
  add disturbance : Subsystem
  updated dPhi : Outport
  wires:
  dPhi/1 -> add disturbance/1(dPhi)
  add disturbance/1(updated dPhi) -> updated dPhi/1

== system Quadrotor_model/Dynamics/Body dynamics/Roll Stability/DisturbancePhi/If Action Subsystem1 ==
  dPhi : Inport
  Action Port : ActionPort  ActionType=else
  updated dPhi : Outport
  wires:
  dPhi/1 -> updated dPhi/1

== system Quadrotor_model/Dynamics/Body dynamics/Yaw Stability/DisturbancePsi/If Action Subsystem ==
  dPsi : Inport
  Action Port : ActionPort  ActionType=then
  add disturbance : Subsystem
  updated dPsi : Outport
  wires:
  dPsi/1 -> add disturbance/1(dPsi)
  add disturbance/1(updated dPsi) -> updated dPsi/1

== system Quadrotor_model/Dynamics/Body dynamics/Yaw Stability/DisturbancePsi/If Action Subsystem1 ==
  dPsi : Inport
  Action Port : ActionPort  ActionType=else
  updated dPsi : Outport
  wires:
  dPsi/1 -> updated dPsi/1

== system Quadrotor_model/Dynamics/Body dynamics/Pitch Stability/DisturbanceTheta/If Action Subsystem/add disturbance ==
  dTheta : Inport
  Subtract : Sum  Inputs=-+
  "vwind " : Subsystem
  updated dTheta : Outport
  wires:
  dTheta/1 -> Subtract/2
  "vwind "/1(vwind) -> Subtract/1
  Subtract/1 -> updated dTheta/1

== system Quadrotor_model/Dynamics/Body dynamics/Position Stability/Disturbancex/If Action Subsystem/add disturbance ==
  dx : Inport
  Subtract : Sum  Inputs=-+
  "vwind " : Subsystem
  updated dx : Outport
  wires:
  dx/1 -> Subtract/2
  "vwind "/1(vwind) -> Subtract/1
  Subtract/1 -> updated dx/1

== system Quadrotor_model/Dynamics/Body dynamics/Position Stability/Disturbancey/If Action Subsystem/add disturbance ==
  dy : Inport
  Subtract : Sum  Inputs=-+
  "vwind " : Subsystem
  updated dy : Outport
  wires:
  dy/1 -> Subtract/2
  "vwind "/1(vwind) -> Subtract/1
  Subtract/1 -> updated dy/1

== system Quadrotor_model/Dynamics/Body dynamics/Position Stability/Disturbancez/If Action Subsystem/add disturbance ==
  dz : Inport
  Subtract : Sum  Inputs=-+
  "vwind " : Subsystem
  updated dz : Outport
  wires:
  dz/1 -> Subtract/2
  "vwind "/1(vwind) -> Subtract/1
  Subtract/1 -> updated dz/1

== system Quadrotor_model/Dynamics/Body dynamics/Roll Stability/DisturbancePhi/If Action Subsystem/add disturbance ==
  dPhi : Inport
  Subtract : Sum  Inputs=-+
  "vwind " : Subsystem
  updated dPhi : Outport
  wires:
  dPhi/1 -> Subtract/2
  "vwind "/1(vwind) -> Subtract/1
  Subtract/1 -> updated dPhi/1

== system Quadrotor_model/Dynamics/Body dynamics/Yaw Stability/DisturbancePsi/If Action Subsystem/add disturbance ==
  dPsi : Inport
  Subtract : Sum  Inputs=-+
  "vwind " : Subsystem
  updated dPsi : Outport
  wires:
  dPsi/1 -> Subtract/2
  "vwind "/1(vwind) -> Subtract/1
  Subtract/1 -> updated dPsi/1

== system Quadrotor_model/Dynamics/Body dynamics/Pitch Stability/DisturbanceTheta/If Action Subsystem/add disturbance/vwind  ==
  Signal Builder : Subsystem  Tag=STV Subsys  LoadFcn=sigbuilder_block('load');  StartFcn=sigbuilder_block('start');  StopFcn=sigbuilder_block('stop');  ClipboardFcn=sigbuilder_block('clipboard');  mask(Sigbuilder block){tuvar=[0:10]}
      mask help: Simulink:masks:SigbuilderBlock_MD
      mask init:
      | if ~strcmp(get_param(bdroot(gcbh),'SimulationStatus'),'stopped') tuvar = sigbuilder_block('maskInit'); end
      settings: CopyFcn=sigbuilder_block('copy');  DeleteFcn=sigbuilder_block('delete');  ModelCloseFcn=sigbuilder_block('modelClose');  PreSaveFcn=sigbuilder_block('preSave');  PauseFcn=sigbuilder_block('pause');  ContinueFcn=sigbuilder_block('continue');  NameChangeFcn=sigbuilder_block('namechange');  OpenFcn=sigbuilder_block('open',[437.6 199.2 550.4 400 ]);  CloseFcn=sigbuilder_block('close');
      mask Display: plot(0, 0, 100, 100,[2, 2, 32, 32, 2], [68, 8, 8, 68, 68],[32, 2], [38, 38], [32, 19, 2],[53, 60, 44], [32, 17, 17, 2],[16, 16, 31, 31]);txt = getActiveGroup(gcbh);text(2, 100, txt,'verticalAlignment', 'top');
  vwind : Outport
  wires:
  Signal Builder/1(Signal 2) -> vwind/1

== system Quadrotor_model/Dynamics/Body dynamics/Position Stability/Disturbancex/If Action Subsystem/add disturbance/vwind  ==
  Signal Builder : Subsystem  Tag=STV Subsys  LoadFcn=sigbuilder_block('load');  StartFcn=sigbuilder_block('start');  StopFcn=sigbuilder_block('stop');  ClipboardFcn=sigbuilder_block('clipboard');  mask(Sigbuilder block){tuvar=[0:10]}
      mask help: Simulink:masks:SigbuilderBlock_MD
      mask init:
      | if ~strcmp(get_param(bdroot(gcbh),'SimulationStatus'),'stopped') tuvar = sigbuilder_block('maskInit'); end
      settings: CopyFcn=sigbuilder_block('copy');  DeleteFcn=sigbuilder_block('delete');  ModelCloseFcn=sigbuilder_block('modelClose');  PreSaveFcn=sigbuilder_block('preSave');  PauseFcn=sigbuilder_block('pause');  ContinueFcn=sigbuilder_block('continue');  NameChangeFcn=sigbuilder_block('namechange');  OpenFcn=sigbuilder_block('open',[394.2 102 550.8 400.2 ]);  CloseFcn=sigbuilder_block('close');
      mask Display: plot(0, 0, 100, 100,[2, 2, 32, 32, 2], [68, 8, 8, 68, 68],[32, 2], [38, 38], [32, 19, 2],[53, 60, 44], [32, 17, 17, 2],[16, 16, 31, 31]);txt = getActiveGroup(gcbh);text(2, 100, txt,'verticalAlignment', 'top');
  vwind : Outport
  wires:
  Signal Builder/1(Signal 1) -> vwind/1

== system Quadrotor_model/Dynamics/Body dynamics/Position Stability/Disturbancey/If Action Subsystem/add disturbance/vwind  ==
  Signal Builder : Subsystem  Tag=STV Subsys  LoadFcn=sigbuilder_block('load');  StartFcn=sigbuilder_block('start');  StopFcn=sigbuilder_block('stop');  ClipboardFcn=sigbuilder_block('clipboard');  mask(Sigbuilder block){tuvar=[0:10]}
      mask help: Simulink:masks:SigbuilderBlock_MD
      mask init:
      | if ~strcmp(get_param(bdroot(gcbh),'SimulationStatus'),'stopped') tuvar = sigbuilder_block('maskInit'); end
      settings: CopyFcn=sigbuilder_block('copy');  DeleteFcn=sigbuilder_block('delete');  ModelCloseFcn=sigbuilder_block('modelClose');  PreSaveFcn=sigbuilder_block('preSave');  PauseFcn=sigbuilder_block('pause');  ContinueFcn=sigbuilder_block('continue');  NameChangeFcn=sigbuilder_block('namechange');  OpenFcn=sigbuilder_block('open',[394.2 102 550.8 400.2 ]);  CloseFcn=sigbuilder_block('close');
      mask Display: plot(0, 0, 100, 100,[2, 2, 32, 32, 2], [68, 8, 8, 68, 68],[32, 2], [38, 38], [32, 19, 2],[53, 60, 44], [32, 17, 17, 2],[16, 16, 31, 31]);txt = getActiveGroup(gcbh);text(2, 100, txt,'verticalAlignment', 'top');
  vwind : Outport
  wires:
  Signal Builder/1(Signal 1) -> vwind/1

== system Quadrotor_model/Dynamics/Body dynamics/Position Stability/Disturbancez/If Action Subsystem/add disturbance/vwind  ==
  Signal Builder : Subsystem  Tag=STV Subsys  LoadFcn=sigbuilder_block('load');  StartFcn=sigbuilder_block('start');  StopFcn=sigbuilder_block('stop');  ClipboardFcn=sigbuilder_block('clipboard');  mask(Sigbuilder block){tuvar=[0:10]}
      mask help: Simulink:masks:SigbuilderBlock_MD
      mask init:
      | if ~strcmp(get_param(bdroot(gcbh),'SimulationStatus'),'stopped') tuvar = sigbuilder_block('maskInit'); end
      settings: CopyFcn=sigbuilder_block('copy');  DeleteFcn=sigbuilder_block('delete');  ModelCloseFcn=sigbuilder_block('modelClose');  PreSaveFcn=sigbuilder_block('preSave');  PauseFcn=sigbuilder_block('pause');  ContinueFcn=sigbuilder_block('continue');  NameChangeFcn=sigbuilder_block('namechange');  OpenFcn=sigbuilder_block('open',[295.2 65.4 595.2 493.8 ]);  CloseFcn=sigbuilder_block('close');
      mask Display: plot(0, 0, 100, 100,[2, 2, 32, 32, 2], [68, 8, 8, 68, 68],[32, 2], [38, 38], [32, 19, 2],[53, 60, 44], [32, 17, 17, 2],[16, 16, 31, 31]);txt = getActiveGroup(gcbh);text(2, 100, txt,'verticalAlignment', 'top');
  vwind : Outport
  wires:
  Signal Builder/1(Signal 2) -> vwind/1

== system Quadrotor_model/Dynamics/Body dynamics/Roll Stability/DisturbancePhi/If Action Subsystem/add disturbance/vwind  ==
  Signal Builder : Subsystem  Tag=STV Subsys  LoadFcn=sigbuilder_block('load');  StartFcn=sigbuilder_block('start');  StopFcn=sigbuilder_block('stop');  ClipboardFcn=sigbuilder_block('clipboard');  mask(Sigbuilder block){tuvar=[0:10]}
      mask help: Simulink:masks:SigbuilderBlock_MD
      mask init:
      | if ~strcmp(get_param(bdroot(gcbh),'SimulationStatus'),'stopped') tuvar = sigbuilder_block('maskInit'); end
      settings: CopyFcn=sigbuilder_block('copy');  DeleteFcn=sigbuilder_block('delete');  ModelCloseFcn=sigbuilder_block('modelClose');  PreSaveFcn=sigbuilder_block('preSave');  PauseFcn=sigbuilder_block('pause');  ContinueFcn=sigbuilder_block('continue');  NameChangeFcn=sigbuilder_block('namechange');  OpenFcn=sigbuilder_block('open',[432 80.25 565.5 403.5 ]);  CloseFcn=sigbuilder_block('close');
      mask Display: plot(0, 0, 100, 100,[2, 2, 32, 32, 2], [68, 8, 8, 68, 68],[32, 2], [38, 38], [32, 19, 2],[53, 60, 44], [32, 17, 17, 2],[16, 16, 31, 31]);txt = getActiveGroup(gcbh);text(2, 100, txt,'verticalAlignment', 'top');
  vwind : Outport
  wires:
  Signal Builder/1(Signal 2) -> vwind/1

== system Quadrotor_model/Dynamics/Body dynamics/Yaw Stability/DisturbancePsi/If Action Subsystem/add disturbance/vwind  ==
  Signal Builder : Subsystem  Tag=STV Subsys  LoadFcn=sigbuilder_block('load');  StartFcn=sigbuilder_block('start');  StopFcn=sigbuilder_block('stop');  ClipboardFcn=sigbuilder_block('clipboard');  mask(Sigbuilder block){tuvar=[0:10]}
      mask help: Simulink:masks:SigbuilderBlock_MD
      mask init:
      | if ~strcmp(get_param(bdroot(gcbh),'SimulationStatus'),'stopped') tuvar = sigbuilder_block('maskInit'); end
      settings: CopyFcn=sigbuilder_block('copy');  DeleteFcn=sigbuilder_block('delete');  ModelCloseFcn=sigbuilder_block('modelClose');  PreSaveFcn=sigbuilder_block('preSave');  PauseFcn=sigbuilder_block('pause');  ContinueFcn=sigbuilder_block('continue');  NameChangeFcn=sigbuilder_block('namechange');  OpenFcn=sigbuilder_block('open',[437.6 199.2 550.4 400 ]);  CloseFcn=sigbuilder_block('close');
      mask Display: plot(0, 0, 100, 100,[2, 2, 32, 32, 2], [68, 8, 8, 68, 68],[32, 2], [38, 38], [32, 19, 2],[53, 60, 44], [32, 17, 17, 2],[16, 16, 31, 31]);txt = getActiveGroup(gcbh);text(2, 100, txt,'verticalAlignment', 'top');
  vwind : Outport
  wires:
  Signal Builder/1(Signal 2) -> vwind/1

== system Quadrotor_model/Dynamics/Body dynamics/Pitch Stability/DisturbanceTheta/If Action Subsystem/add disturbance/vwind /Signal Builder ==
  Demux : Demux  Tag=STV Demux  Outputs=1
  FromWs : FromWorkspace  Tag=STV FromWs  VariableName=tuvar  SampleTime=0
      SigBuilderData=|
      | common.afterFinalStr = 'Extrapolate'
      | common.sampleTime = 0
      | dataSet.timeRange = [0 20]
      | dataSet.name = 'Group 1'
      | sbobj.Groups.Name = 'Group 1'
      | sbobj.Groups.Signals.Name = 'Signal 2'
      | sbobj.Groups.Signals.XData = [0 0.1 0.2 0.3 0.4 0.5 0.6 0.7 0.8 0.9 1 1.1 1.2 1.3 1.4 1.5 1.6 1.7 1.8 1.9 2 2.1 2.2 2.3 2.4 2.5 2.6 2.7 2.8 2.9 3 3.1 3.2 3.3 3.4 3.5 3.6 3.7 3.8 3.9 4 4.1 4.2 4.3 4.4 4.5 4.6 4.7 4.8 4.9 5 5.1 5.2 5.3 5.4 5.5 5.6 5.7 5.8 5.9 6 6.1 6.2 6.3 6.4 6.5 6.6 6.7 6.8 6.9 7 7.1 7.2 7.3 7.4 7.5 7.6 7.7 7.8 7.9 8 8.1 8.2 8.3 8.4 8.5 8.6 8.7 8.8 8.9 9 9.1 9.2 9.3 9.4 9.5 9.6 9.7 9.8 9.9 10 10.1 10.2 10.3 10.4 10.5 10.6 10.7 10.8 10.9 11 11.1 11.2 11.3 11.4 11.5 11.6 11.7 11.8 11.9 12 12.1 12.2 12.3 12.4 12.5 12.6 12.7 12.8 12.9 13 13.1 13.2 13.3 13.4 13.5 13.6 13.7 13.8 13.9 14 14.1 14.2 14.3 14.4 14.5 14.6 14.7 14.8 14.9 15 15.1 15.2 15.3 15.4 15.5 15.6 15.7 15.8 15.9 16 16.1 16.2 16.3 16.4 16.5 16.6 16.7 16.8 16.9 17 17.1 17.2 17.3 17.4 17.5 17.6 17.7 17.8 17.9 18 18.1 18.2 18.3 18.4 18.5 18.6 18.7 18.8 18.9 19 19.1 19.2 19.3 19.4 19.5 19.6 19.7 19.8 19.9 20]
      | sbobj.Groups.Signals.YData = [0.383023912781 0.412035378112 0.405492550516 -0.363780750881 -0.599272040042 -0.589588991418 0.853540834064 -1.85300807142 -0.207303159648 0.27037820269 -0.652771012059 0.477227285008 ... (201 elements, 1x201)]
      | sbobj.Groups.TimeRange = [0 20]
  Signal 2 : Outport  Tag=STV Outport
  wires:
  FromWs/1 -> Demux/1
  Demux/1 -> Signal 2/1

== system Quadrotor_model/Dynamics/Body dynamics/Position Stability/Disturbancex/If Action Subsystem/add disturbance/vwind /Signal Builder ==
  Demux : Demux  Tag=STV Demux  Outputs=1
  FromWs : FromWorkspace  Tag=STV FromWs  VariableName=tuvar  SampleTime=0
      SigBuilderData=|
      | common.afterFinalStr = 'Extrapolate'
      | common.sampleTime = 0
      | dataSet.timeRange = [0 10]
      | dataSet.name = 'Group 1'
      | sbobj.Groups.Name = 'Group 1'
      | sbobj.Groups.Signals.Name = 'Signal 1'
      | sbobj.Groups.Signals.XData = [0 2 2 2.001 10]
      | sbobj.Groups.Signals.YData = [0 0 10000 0 0]
  Signal 1 : Outport  Tag=STV Outport
  wires:
  Demux/1 -> Signal 1/1
  FromWs/1 -> Demux/1

== system Quadrotor_model/Dynamics/Body dynamics/Position Stability/Disturbancey/If Action Subsystem/add disturbance/vwind /Signal Builder ==
  Demux : Demux  Tag=STV Demux  Outputs=1
  FromWs : FromWorkspace  Tag=STV FromWs  VariableName=tuvar  SampleTime=0
      SigBuilderData=|
      | common.afterFinalStr = 'Extrapolate'
      | common.sampleTime = 0
      | dataSet.timeRange = [0 10]
      | dataSet.name = 'Group 1'
      | sbobj.Groups.Name = 'Group 1'
      | sbobj.Groups.Signals.Name = 'Signal 1'
      | sbobj.Groups.Signals.XData = [0 2 2 2.001 10]
      | sbobj.Groups.Signals.YData = [0 0 10000 0 0]
  Signal 1 : Outport  Tag=STV Outport
  wires:
  Demux/1 -> Signal 1/1
  FromWs/1 -> Demux/1

== system Quadrotor_model/Dynamics/Body dynamics/Position Stability/Disturbancez/If Action Subsystem/add disturbance/vwind /Signal Builder ==
  Demux : Demux  Tag=STV Demux  Outputs=1
  FromWs : FromWorkspace  Tag=STV FromWs  VariableName=tuvar  SampleTime=0
      SigBuilderData=|
      | common.afterFinalStr = 'Extrapolate'
      | common.sampleTime = 0
      | dataSet.timeRange = [0 10]
      | dataSet.name = 'Group 1'
      | sbobj.Groups.Name = 'Group 1'
      | sbobj.Groups.Signals.Name = 'Signal 2'
      | sbobj.Groups.Signals.XData = [0 4 4 5 5 10]
      | sbobj.Groups.Signals.YData = [0 0 40 40 0 0]
  Signal 2 : Outport  Tag=STV Outport
  wires:
  FromWs/1 -> Demux/1
  Demux/1 -> Signal 2/1

== system Quadrotor_model/Dynamics/Body dynamics/Roll Stability/DisturbancePhi/If Action Subsystem/add disturbance/vwind /Signal Builder ==
  Demux : Demux  Tag=STV Demux  Outputs=1
  FromWs : FromWorkspace  Tag=STV FromWs  VariableName=tuvar  SampleTime=0
      SigBuilderData=|
      | common.afterFinalStr = 'Extrapolate'
      | common.sampleTime = 0
      | dataSet.timeRange = [0 20]
      | dataSet.name = 'Group 1'
      | sbobj.Groups.Name = 'Group 1'
      | sbobj.Groups.Signals.Name = 'Signal 2'
      | sbobj.Groups.Signals.XData = [0 0.1 0.2 0.3 0.4 0.5 0.6 0.7 0.8 0.9 1 1.1 1.2 1.3 1.4 1.5 1.6 1.7 1.8 1.9 2 2.1 2.2 2.3 2.4 2.5 2.6 2.7 2.8 2.9 3 3.1 3.2 3.3 3.4 3.5 3.6 3.7 3.8 3.9 4 4.1 4.2 4.3 4.4 4.5 4.6 4.7 4.8 4.9 5 5.1 5.2 5.3 5.4 5.5 5.6 5.7 5.8 5.9 6 6.1 6.2 6.3 6.4 6.5 6.6 6.7 6.8 6.9 7 7.1 7.2 7.3 7.4 7.5 7.6 7.7 7.8 7.9 8 8.1 8.2 8.3 8.4 8.5 8.6 8.7 8.8 8.9 9 9.1 9.2 9.3 9.4 9.5 9.6 9.7 9.8 9.9 10 10.1 10.2 10.3 10.4 10.5 10.6 10.7 10.8 10.9 11 11.1 11.2 11.3 11.4 11.5 11.6 11.7 11.8 11.9 12 12.1 12.2 12.3 12.4 12.5 12.6 12.7 12.8 12.9 13 13.1 13.2 13.3 13.4 13.5 13.6 13.7 13.8 13.9 14 14.1 14.2 14.3 14.4 14.5 14.6 14.7 14.8 14.9 15 15.1 15.2 15.3 15.4 15.5 15.6 15.7 15.8 15.9 16 16.1 16.2 16.3 16.4 16.5 16.6 16.7 16.8 16.9 17 17.1 17.2 17.3 17.4 17.5 17.6 17.7 17.8 17.9 18 18.1 18.2 18.3 18.4 18.5 18.6 18.7 18.8 18.9 19 19.1 19.2 19.3 19.4 19.5 19.6 19.7 19.8 19.9 20]
      | sbobj.Groups.Signals.YData = [-0.0957388204404 3.40266930855 -1.01942342553 -0.00570992028864 1.83973415961 0.299617465266 2.80986689135 2.06824307914 0.583140577542 -1.55539707662 1.13339219508 -2.76524231896 ... (201 elements, 1x201)]
      | sbobj.Groups.TimeRange = [0 20]
  Signal 2 : Outport  Tag=STV Outport
  wires:
  FromWs/1 -> Demux/1
  Demux/1 -> Signal 2/1

== system Quadrotor_model/Dynamics/Body dynamics/Yaw Stability/DisturbancePsi/If Action Subsystem/add disturbance/vwind /Signal Builder ==
  Demux : Demux  Tag=STV Demux  Outputs=1
  FromWs : FromWorkspace  Tag=STV FromWs  VariableName=tuvar  SampleTime=0
      SigBuilderData=|
      | common.afterFinalStr = 'Extrapolate'
      | common.sampleTime = 0
      | dataSet.timeRange = [0 10]
      | dataSet.name = 'Group 1'
      | sbobj.Groups.Name = 'Group 1'
      | sbobj.Groups.Signals.Name = 'Signal 2'
      | sbobj.Groups.Signals.XData = [0 2 2 3 3 10]
      | sbobj.Groups.Signals.YData = [0 0 500 500 0 0]
  Signal 2 : Outport  Tag=STV Outport
  wires:
  FromWs/1 -> Demux/1
  Demux/1 -> Signal 2/1

== matlab function Quadrotor_model/Controller/calculateU ==
  data: X input; U output; dX input; Xdes input; Xdesdot input; s input; Omega input
function U  = fcn(X,dX,Xdes,Xdesdot,s,Omega)

U    = zeros(4,1);
sats = zeros(4,1);

W = Omega;

p = load('QuadrotorConstants'); % Load quadrotor constants
t = load('TuningParameters');   % Load tuning parameters

for i = 1:length(s)
    sats(i) = tanh(s(i));
end

U(1,1) = p.m/cos(X(7))/cos(X(9))*(Xdesdot(6)+p.ga+t.lambda(1)*(Xdes(6)-X(6))+t.lambdai(1)*(Xdes(5)-X(5))+t.K(1)*sats(1)+t.eta(1)*s(1));
U(2,1) = (p.Ixx/p.L)*(Xdesdot(8)-((p.Izz-p.Ixx)/(p.Iyy))*X(8)*X(12)+(p.Jr/p.Ixx)*X(10)*W+t.lambda(2)*(Xdes(8)-X(8))+t.lambdai(2)*(Xdes(7)-X(7))+t.K(2)*sats(2)+t.eta(2)*s(2));
U(3,1) = (p.Ixx/p.L)*(Xdesdot(10)-((p.Izz-p.Ixx)/(p.Iyy))*X(8)*X(12)+(p.Jr/p.Ixx)*X(8)*W+t.lambda(3)*(Xdes(10)-X(10))+t.lambdai(3)*(Xdes(9)-X(9))+t.K(3)*sats(3)+t.eta(3)*s(3));
U(4,1) = p.Izz*(Xdesdot(12)-((p.Ixx-p.Iyy)/(p.Izz))*X(8)*X(10)+t.lambda(4)*(Xdes(12)-X(12))+t.lambdai(4)*(Xdes(11)-X(11))+t.K(4)*sats(4)+t.eta(4)*s(4));

% U(1,1) = p.m/cos(X(7))/cos(X(9))*(Xdesdot(6)+p.ga+t.lambda(1)*(Xdes(6)-X(6))+t.lambdai(1)*(Xdes(5)-X(5))+t.K(1)*sats(1)+t.eta(1)*s(1));
% U(2,1) = (p.Ixx/p.L)*(Xdesdot(8)-((p.Izz-p.Ixx)/(p.Iyy))*X(8)*X(12)+(p.Jr/p.Ixx)*X(10)*W+t.lambda(2)*(Xdes(8)-X(8))+t.lambdai(2)*(Xdes(7)-X(7))+t.K(2)*sats(2)+t.eta(2)*s(2)+t.lambda(5)*(Xdes(2)-X(2))+t.lambdai(5)*(Xdes(1)-X(1))+(Xdesdot(2)-(cos(X(7))*sin(X(9))*cos(X(11))+sin(X(7))*sin(X(11))))*U(1,1)/p.m);
% U(3,1) = (p.Ixx/p.L)*(Xdesdot(10)-((p.Izz-p.Ixx)/(p.Iyy))*X(8)*X(12)+(p.Jr/p.Ixx)*X(8)*W+t.lambda(3)*(Xdes(10)-X(10))+t.lambdai(3)*(Xdes(9)-X(9))+t.K(3)*sats(3)+t.eta(3)*s(3)+t.lambda(6)*(Xdes(4)-X(4))+t.lambdai(6)*(Xdes(3)-X(3))+(Xdesdot(4)-(cos(X(7))*sin(X(9))*sin(X(11))-sin(X(7))*cos(X(11))))*U(1,1)/p.m);
% U(4,1) = p.Izz*(Xdesdot(12)-((p.Ixx-p.Iyy)/(p.Izz))*X(8)*X(10)+t.lambda(4)*(Xdes(12)-X(12))+t.lambdai(4)*(Xdes(11)-X(11))+t.K(4)*sats(4)+t.eta(4)*s(4));

end

== matlab function Quadrotor_model/Correct for Singularities/Check for singularity in phi, theta/Singularity in phi/CorrectPhi ==
  data: X input; newX output; XDes input
function newX = fcn(X, XDes)

% Initialize the variables
newX   = X;
newphi = 0;
err    = 0;
% Unpack the state
phi    = X(7);
phiDes = XDes(7);
% Tolerance
tol    = 0.25;

if abs(phi-pi/2) < tol
    err = phiDes-phi;
    if err>=0
        newphi = phi+2*tol;
    elseif err<0
        newphi = phi - 2*tol;
    end
    
elseif abs(phi-3*pi/2) < tol
    err = phiDes-phi;
    if err>=0
        newphi = phi+2*tol;
    elseif err<0
        newphi = phi - 2*tol;
    end
else
    newphi = phi;
end

newX(7) = newphi;


end

== matlab function Quadrotor_model/Controller/findVolts/MATLAB Function ==
  data: U input; Omegas output
function Omegas = fcn(U)

% initialize memory for omega
Omegas = zeros(4,1);

% coefficients
bb = 2.6846e-07;
dd = 2.4481e-08;

% linear system matrix
A = [bb bb bb bb; 0 -bb 0 bb; -bb 0 bb 0; -dd dd -dd dd];

% Omegas = A\U;
% 
% for i = 1:length(Omegas)
%     Omegas(i) = real(Omegas(i));
% end
% 
% Omegas = sqrt(Omegas);


% square root all of the omega values
Omegas = sqrt((A\U).*sign(A\U));
% if sum(imag(complex(A\U))) ~= 0
% Omegas = sqrt(complex(real(A\U),imag(A\U)));%.*sign(A\U));
% else
% Omegas = sqrt(A\U);%.*sign(A\U));
% end
end

== matlab function Quadrotor_model/Correct for Singularities/Check for singularity in phi, theta/Singularity in theta/CorrectTheta ==
  data: X input; newX output; XDes input
function newX = fcn(X, XDes)
newX = X;
newtheta = 0;
err = 0;
theta = X(9);
thetaD = XDes(9);
tol = 0.25;

if abs(theta-pi/2) < tol
    err = thetaD-theta;
    if err>=0
        newtheta = theta+2*tol;
    elseif err<0
        newtheta = theta - 2*tol;
    end
    
elseif abs(theta-3*pi/2) < tol
    err = thetaD-theta;
    if err>=0
        newtheta = theta+2*tol;
    elseif err<0
        newtheta = theta - 2*tol;
    end
else
    newtheta = theta;
end

newX(9) = newtheta;


end
